simulink model "dummy"  (R2025b)
settings: Solver=VariableStepAuto  StartTime=0.0  StopTime=119  RelTol=1e-3
values from neighbouring files (symbols this model uses):
  Ts = 0.01    [generate_random_trajectories.m]    (also in main.m; main_posture_regulation.m; main_unicycle_tracking.m; random_trajectories.mat)
settings Model: Creator=nyanklc  LastModifiedBy=nyanklc

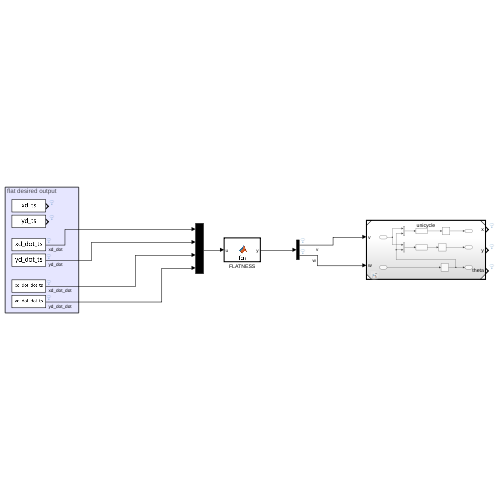
[thumbnail: Simulink's stored preview of the top-level diagram]
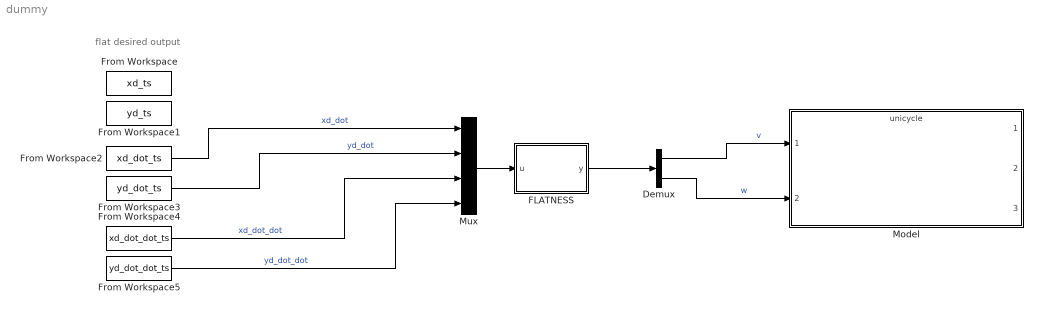
== system dummy ==
  note: flat desired output
  Demux : Demux  Outputs=2
  FLATNESS : MATLAB Function  TreatAsAtomicUnit=on
  From Workspace : FromWorkspace  VariableName=xd_ts  SampleTime=Ts  OutputAfterFinalValue=Holding final value
  From Workspace1 : FromWorkspace  VariableName=yd_ts  SampleTime=Ts  OutputAfterFinalValue=Holding final value
  From Workspace2 : FromWorkspace  VariableName=xd_dot_ts  SampleTime=Ts  OutputAfterFinalValue=Holding final value
  From Workspace3 : FromWorkspace  VariableName=yd_dot_ts  SampleTime=Ts  OutputAfterFinalValue=Holding final value
  From Workspace4 : FromWorkspace  VariableName=xd_dot_dot_ts  SampleTime=Ts  OutputAfterFinalValue=Holding final value
  From Workspace5 : FromWorkspace  VariableName=yd_dot_dot_ts  SampleTime=Ts  OutputAfterFinalValue=Holding final value
  Model : ModelReference  ModelNameDialog=unicycle.slx  SimulationMode=Normal  ModelReferenceVersion=1.7
  Mux : Mux
  wires:
  FLATNESS/1(y) -> Demux/1
  Demux/1 -> Model/1  "v"
  Mux/1 -> FLATNESS/1(u)
  Demux/2 -> Model/2  "w"
  From Workspace2/1 -> Mux/1  "xd_dot"
  From Workspace3/1 -> Mux/2  "yd_dot"
  From Workspace4/1 -> Mux/3  "xd_dot_dot"
  From Workspace5/1 -> Mux/4  "yd_dot_dot"

== matlab function dummy/FLATNESS ==
  data: u input; y output
function y = fcn(u)

xd_dot = u(1);
yd_dot= u(2);
xd_dot_dot = u(3);
yd_dot_dot= u(4);

v = sqrt(xd_dot^2 + yd_dot^2);
w = (xd_dot*yd_dot_dot - xd_dot_dot*yd_dot) / (xd_dot^2 + yd_dot^2);

y = [v; w];
